simulink model "stuPlutoRx"  (R2019b)
settings: Solver=VariableStepAuto  StartTime=0.0  StopTime=5  RelTol=1e-3
undefined symbols (not defined in the file): designMultirateFIR, fdesignblkfcn, Fs, gcbh, ip, usb
libraries: dspfdesign x2, plutoradiolib x1, dspmlti4 x1
settings Model: Creator=dm  LastModifiedBy=LYM
settings DebuggingCC: SFMachineParentedDataDiag=error

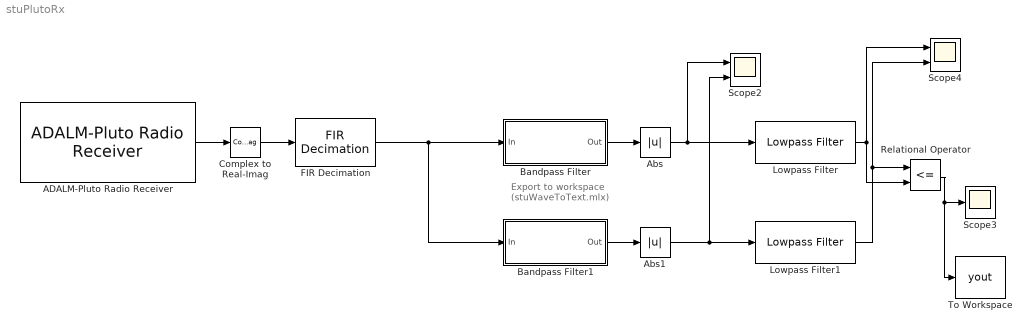
== system stuPlutoRx ==
  note: Export to workspace
      | (stuWaveToText.mlx)
  ADALM-Pluto Radio Receiver : plutoradiolib/ADALM-Pluto Radio Receiver  RadioID=usb:0  uri=ip:10.0.0.200  CenterFrequencySource=Dialog  CenterFrequency=915.432e6  GainSource=AGC Slow Attack  GainSourceBlock=AGC Slow Attack  Gain=10  ChannelMapping=1  BasebandSampleRate=1e6  OutputDataType=double  SamplesPerFrame=1e4  OverflowOutputPort=off  EnableBurstMode=off  NumFramesInBurst=1  ShowAdvancedProperties=off  UseCustomFilter=off  filtPathRates=[737280000 11520000 3840000 1920000 960000 240000]  filtCoefficients=[-192 82 85 -215 228 -102 -110 290 -318 145 160 -426 471 -215 -238 633 -697 318 349 -923 1009 -457 -498 1309 -1423 640 693 -1812 1959 -876 -945 2458 -2647 1180 1268 -3290 3534 -1572 -1688 4375 -4698 2091 2247 -5836 6284 -2807 -3031 7918 -8588 3870 4225 -11182 12324 -5662 -6330 17255 -19735 9507 11312 -33568 43355 -25227 -42139 305542 305542 -42139 -25227 43355 -33568 11312 9507 -19735 17255 -6330 -5662 12324 -11182 4225 3870 -8588 7918 -3031 -2807 6284 -5836 2247 2091 -4698 4375 -1688 -1572 3534 -3290 1268 1180 -2647 2458 -945 -876 1959 -1812 693 640 -1423 1309 -498 -457 1009 -923 349 318 -697 633 -238 -215 471 -426 160 145 -318 290 -110 -102 228 -215 85 82 -192]  filtCoefficientSize=128  filtDecimInterpFactor=4  filtGain=-12  filtRFBandwidth=18000000  filterConfigStruct=struct()  EnableQuadratureCorrection=on  EnableRFDCCorrection=on  EnableBasebandDCCorrection=on  FrequencyCorrection=0  OverrideSampleTime=off  SampleTime=0.02  DataTimeout=Inf  ENSMPinControlMode=None  BISTLoopbackMode=Disabled  BISTToneInject=Disabled  BISTSignalGen=PRBS  BISTToneFreq=Fs/32  BISTToneLevel=0
      settings: SourceProductBaseCode=PLUTO
  Abs : Abs
  Abs1 : Abs
  Bandpass Filter : Subsystem  DialogController=fdesignblkfcn  InitFcn=fdesignblkfcn(gcbh, {'InitFcn'});  mask(Bandpass Filter){}
      mask help: Design a bandpass filter
      settings: CopyFcn=fdesignblkfcn(gcbh, {'CopyFcn'});
      mask Help: helpview(mapfilelocation('dsp'), 'dspbandpassfilter');
      mask Display: disp('Bandpass');
  Bandpass Filter1 : Subsystem  DialogController=fdesignblkfcn  InitFcn=fdesignblkfcn(gcbh, {'InitFcn'});  mask(Bandpass Filter){}
      mask help: Design a bandpass filter
      settings: CopyFcn=fdesignblkfcn(gcbh, {'CopyFcn'});
      mask Help: helpview(mapfilelocation('dsp'), 'dspbandpassfilter');
      mask Display: disp('Bandpass');
  Complex to Real-Imag : ComplexToRealImag  Output=Real
  FIR Decimation : dspmlti4/FIR Decimation  FilterSource=Auto  h=designMultirateFIR(1,2)  D=10  filtStruct=Direct form  FilterObject=FDECIM  InputProcessing=Columns as channels (frame based)  framing=Allow multirate processing  inputOffset=0  outputBufInitCond=0  roundingMode=Floor  overflowMode=off  firstCoeffDataTypeStr=Inherit: Same word length as input  firstCoeffMin=[]  firstCoeffMax=[]  firstCoeffLastDataTypeStr=Inherit: Same word length as input  outputDataTypeStr=Inherit: Same as accumulator  outputMin=[]  outputMax=[]  outputLastDataTypeStr=Inherit: Same as accumulator
  Lowpass Filter : dspfdesign/Lowpass Filter  FilterType=FIR  DesignForMinimumOrder=on  FilterOrder=50  PassbandFrequency=3e3  StopbandFrequency=5e3  PassbandRipple=0.1  StopbandAttenuation=80  InheritSampleRate=off  SampleRate=100000  SimulateUsing=Interpreted execution  roundingMode=Floor  coeffsDataTypeStr=fixdt(1,16)
  Lowpass Filter1 : dspfdesign/Lowpass Filter  FilterType=FIR  DesignForMinimumOrder=on  FilterOrder=50  PassbandFrequency=3e3  StopbandFrequency=5e3  PassbandRipple=0.1  StopbandAttenuation=80  InheritSampleRate=off  SampleRate=100000  SimulateUsing=Interpreted execution  roundingMode=Floor  coeffsDataTypeStr=fixdt(1,16)
  Relational Operator : RelationalOperator  Operator=<=  OutDataTypeStr=boolean  RndMeth=Simplest
  Scope2 : Scope  NumInputPorts=2
  Scope3 : Scope
  Scope4 : Scope  NumInputPorts=2
  To Workspace : ToWorkspace  VariableName=yout  SampleTime=-1
      settings: Save2DSignal=2-D array (concatenate along first dimension)
  wires:
  ADALM-Pluto Radio Receiver/1 -> Complex to Real-Imag/1
  Complex to Real-Imag/1 -> FIR Decimation/1
  Lowpass Filter1/1 -> Scope4/2, Relational Operator/1
  FIR Decimation/1 -> Bandpass Filter1/1(In), Bandpass Filter/1(In)
  Abs1/1 -> Lowpass Filter1/1, Scope2/2
  Lowpass Filter/1 -> Scope4/1, Relational Operator/2
  Abs/1 -> Lowpass Filter/1, Scope2/1
  Relational Operator/1 -> To Workspace/1, Scope3/1
  Bandpass Filter1/1(Out) -> Abs1/1
  Bandpass Filter/1(Out) -> Abs/1

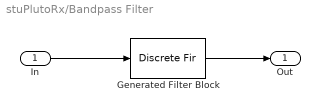
== system stuPlutoRx/Bandpass Filter ==
  In : Inport
  Generated Filter Block : DiscreteFir  Tag=BlockMethodSubSystem  Coefficients=[0.000213316643211492954 -0.000635592453794410288 -0.000504334816704885957 0.000152890060088685907 0.000683606408538445383 0.000248579424616465056 -0.000680141997885299774 -0.000747282976328058918 0.000282298406287287233 0.000989415527253485229 0.000323911083659441648 -0.000773883097237419455 -0.000751848942015291566 0.000235546294066168251 0.000696807402697022672 0.000183969777137975039 -0.000244622470049292407 -6.6809937404982295e-05 -9.27039010097828388e-05 -0.000563604102740889357 -0.000266908725549804319 0.00110248957012071399 0.00142859872360460495 -0.00071634480091262566 -0.00272383781172639552 -0.000970205302235905708 0.00300470271356912929 0.00336310229005259238 -0.00145107527685541839 -0.00504978305627132567 -0.00165744714087356763 0.00466507824366131987 0.0048496681597449123 -0.00193108623293049265 -0.00628479927538761959 -0.0019245617911931702 0.00501316512323349284 0.00482444456623894874 -0.00176448054987879952 -0.00522935432550063455 -0.00143347562138400309 0.00328205415125247969 0.00266055786371592129 -0.000776734639496856573 -0.00154872232965612704 -0.00016050025527768118 -0.000364699792747795535 -0.00124125626778905551 0.000786339591000873072 0.00365205731565671583 0.00146000255896806667 -0.00455371468897758456 -0.00528553142675412639 0.00224000354456285267 0.00794175534982302471 0.00262109157703159035 -0.00707689861096345591 -0.00720316138182876004 0.00271380749744398134 0.00854550000807611197 0.00249860132026514256 -0.00591957703594111519 -0.00517334893656942307 0.00160802456206406695 0.00388574179500333992 0.000735775393665834125 -0.000532700966723424285 0.000932948070219666737 -0.000956522950425980336 -0.0050630388314487438 -0.00218148206799022608 0.00732963026125272189 0.00888180487293543756 -0.00395271426128188455 -0.0144361487161961954 -0.00490552511172325043 0.0137972761103362668 0.014508771921236039 -0.0057049222983547674 -0.0186128635681302168 -0.0056687250889436748 0.01425281835060907 0.0132875643533305627 -0.00455418539535396363 -0.0125563047062762622 -0.00305052405838876365 0.00541697737463453944 0.00245689711817129739 0.00033019149095303655 0.00561432739950365467 0.00326033120203831099 -0.0127844314833018349 -0.0172818508174610135 0.00838129896761286367 0.0330819325881602164 0.0120942505486901757 -0.0365464079267498049 -0.0414128833535119603 0.0176271999577141646 0.0627359640812465563 0.0210594958077986033 -0.059198984364551295 -0.0629505479581709271 0.0253217466594902081 0.0855703108675154034 0.0273813227338298576 -0.0736168108138092331 -0.075025444278933151 0.0289813366709299608 0.0941406662414492196 0.0289813366709299608 -0.075025444278933151 -0.0736168108138092331 0.0273813227338298576 0.0855703108675154034 0.0253217466594902081 -0.0629505479581709271 -0.059198984364551295 0.0210594958077986033 0.0627359640812465563 0.0176271999577141646 -0.0414128833535119603 -0.0365464079267498049 0.0120942505486901757 0.0330819325881602164 0.00838129896761286367 -0.0172818508174610135 -0.0127844314833018349 0.00326033120203831099 0.00561432739950365467 0.00033019149095303655 0.00245689711817129739 0.00541697737463453944 -0.00305052405838876365 -0.0125563047062762622 -0.00455418539535396363 0.0132875643533305627 0.01425281835060907 -0.0056687250889436748 -0.0186128635681302168 -0.0057049222983547674 0.014508771921236039 0.0137972761103362668 -0.00490552511172325043 -0.0144361487161961954 -0.00395271426128188455 0.00888180487293543756 0.00732963026125272189 -0.00218148206799022608 -0.0050630388314487438 -0.000956522950425980336 0.000932948070219666737 -0.000532700966723424285 0.000735775393665834125 0.00388574179500333992 0.00160802456206406695 -0.00517334893656942307 -0.00591957703594111519 0.00249860132026514256 0.00854550000807611197 0.00271380749744398134 -0.00720316138182876004 -0.00707689861096345591 0.00262109157703159035 0.00794175534982302471 0.00224000354456285267 -0.00528553142675412639 -0.00455371468897758456 0.00146000255896806667 0.00365205731565671583 0.000786339591000873072 ...(+1153 chars)]  InputProcessing=Columns as channels (frame based)
  Out : Outport  VectorParamsAs1DForOutWhenUnconnected=off
  wires:
  In/1 -> Generated Filter Block/1
  Generated Filter Block/1 -> Out/1

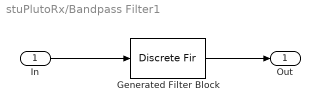
== system stuPlutoRx/Bandpass Filter1 ==
  In : Inport
  Generated Filter Block : DiscreteFir  Tag=BlockMethodSubSystem  Coefficients=[0.000611513415512140806 0.00020121591073089546 -4.0904644584845867e-05 -0.000414901041852736355 -0.000755749267473578663 -0.00086948818547137065 -0.000636451574687462666 -9.29099999592013942e-05 0.000558793033910233157 0.00103605340162417738 0.0011102457837702921 0.000732458861958381799 7.39795349236168536e-05 -0.00056061876071524506 -0.000888862721604435414 -0.000809352593160481181 -0.000454508416373289802 -0.000107945887166894226 -1.84568644530254118e-05 -0.000223388844762660251 -0.000496865201347149871 -0.0004723163523700353 0.000109680596993834705 0.0011715050384494411 0.00224203085357805535 0.00264331927877294341 0.00185843715637081701 -0.000111543584711229276 -0.00261227072505724458 -0.00454787170488927042 -0.00487715838989165231 -0.00316497072536967277 0.00010447579249313289 0.00365276410740988586 0.0059530576249291348 0.00595043332919849462 0.00359546849874769906 -9.82228550514298564e-05 -0.00352460875838916075 -0.00526117468513600389 -0.0047511309638485974 -0.00253490571753841806 9.40870163710387161e-05 0.00182085255015956263 0.00202260609296810081 0.00106465220815494589 9.51407152178563621e-06 -9.28828215981797583e-05 0.00108363297706563473 0.0028626345929452816 0.00391490339777518861 0.0030639755671375505 9.06388201201230531e-05 -0.00395563931037880637 -0.0071731755071177683 -0.00777650426071234066 -0.00510289350801655054 -8.25303982483716015e-05 0.005132828129387354 0.00822716326920393259 0.00790893256412527473 0.00457523164198633207 6.65412449467829483e-05 -0.00336942140101691634 -0.00432764468202274759 -0.00299197462448727493 -0.000930826209470207396 -4.41159118781250456e-05 -0.00127662032805990369 -0.00388683724458574378 -0.00577093548447936942 -0.00472991987569877474 2.14240169357010277e-05 0.00701981283235598823 0.0129918695986975564 0.0144603084728992335 0.0097077921949961718 -5.34361836243557597e-06 -0.0107468616616318603 -0.0177158004848091202 -0.0176622419352315749 -0.0106271227746427294 2.13040097606000817e-07 0.00922341835471719718 0.0130864492908872414 0.0107715287591817806 0.00493129516054016236 -5.47973466491187902e-06 -0.000643608274927515048 0.00308569761024766629 0.00760003959042735919 0.00770622377973523634 1.52239004385158229e-05 -0.0142049993910912595 -0.0285878537152104359 -0.0343099032759073622 -0.0247811678013552424 -2.13992045513863166e-05 0.031802622039223058 0.0569864101358219452 0.0622770531476080358 0.0415785498759416103 1.8906228784540749e-05 -0.0469864505825314249 -0.0797450957518917036 -0.0829202713208838649 -0.0528527405570773309 -7.59687512593039405e-06 0.054882452279927621 0.0894773538261672552 0.0894773538261672552 0.054882452279927621 -7.59687512593039405e-06 -0.0528527405570773309 -0.0829202713208838649 -0.0797450957518917036 -0.0469864505825314249 1.8906228784540749e-05 0.0415785498759416103 0.0622770531476080358 0.0569864101358219452 0.031802622039223058 -2.13992045513863166e-05 -0.0247811678013552424 -0.0343099032759073622 -0.0285878537152104359 -0.0142049993910912595 1.52239004385158229e-05 0.00770622377973523634 0.00760003959042735919 0.00308569761024766629 -0.000643608274927515048 -5.47973466491187902e-06 0.00493129516054016236 0.0107715287591817806 0.0130864492908872414 0.00922341835471719718 2.13040097606000817e-07 -0.0106271227746427294 -0.0176622419352315749 -0.0177158004848091202 -0.0107468616616318603 -5.34361836243557597e-06 0.0097077921949961718 0.0144603084728992335 0.0129918695986975564 0.00701981283235598823 2.14240169357010277e-05 -0.00472991987569877474 -0.00577093548447936942 -0.00388683724458574378 -0.00127662032805990369 -4.41159118781250456e-05 -0.000930826209470207396 -0.00299197462448727493 -0.00432764468202274759 -0.00336942140101691634 6.65412449467829483e-05 0.00457523164198633207 0.00790893256412527473 0.00822716326920393259 0.005132828129387354 -8.25303982483716015e-05 -0.00510289350801655054 -0.00777650426071234066 -0.0071731755071177683 -0.00395563931037880637 9.06388201201230531e-05 0.0030639755671375505 0.00391490339777518861 ...(+1191 chars)]  InputProcessing=Columns as channels (frame based)
  Out : Outport  VectorParamsAs1DForOutWhenUnconnected=off
  wires:
  In/1 -> Generated Filter Block/1
  Generated Filter Block/1 -> Out/1
